simulink model "model"  (R2022a)
settings: Solver=VariableStepAuto  StartTime=0.0  StopTime=5000  RelTol=1e-3
values from neighbouring files (symbols this model uses):
  AIR_minus_delay = round(0.6/Ts)    [parameters.m]    (also in parameters.mat = 3)
  AIR_plus_delay = round(0.6/Ts)    [parameters.m]    (also in parameters.mat = 3)
  C_index = 3    [parameters.m]    (also in parameters.mat)
  C_r = 6.6    [parameters.m]    (also in parameters.mat)
  Cap_det = -1e-7    (= -1e-07)    [parameters.m]    (also in parameters.mat)
  cCap = awgn(cCap, -60)    [parameters.m]    (also in parameters.mat = [22398.4850451 24107.592632 23578.1567815 22820.4652341 2372)
  cell_count = 126    [parameters.m]    (also in parameters.mat)
  cQur = cCap / 2    [parameters.m]    (also in parameters.mat = [11880 11880 11880 11880 11880 11880 11880 11880 11880 11880)
  cTmp = 20*ones(60, 1)    [parameters.m]    (also in parameters.mat = [20 20 20 20 20 20 20 20 20 20 20 20 ... (60 elements, 60x1))
  I_CV = 1    [parameters.m]    (also in parameters.mat)
  ocv = ocv_LUT    [parameters.m]    (also in parameters.mat = [0 2.99808472822 3.29015678206 3.51449858493 3.66802196423 3)
  precharge_delay = round(0.3/Ts)    [parameters.m]    (also in parameters.mat = 1)
  Q_index = 2    [parameters.m]    (also in parameters.mat)
  R_short = 33    [parameters.m]    (also in parameters.mat)
  Rp = Rp_LUT    [parameters.m]    (also in parameters.mat = [0.0013284973182 0.00132849731829 0.00133071540687 0.0013310)
  Rs = Rs_LUT    [parameters.m]    (also in parameters.mat = [0.0044622496006 0.00446224960062 0.00395928973129 0.0036572)
  soc = soc_LUT    [parameters.m]    (also in parameters.mat = [0 0.01 0.0909090909091 0.181818181818 0.272727272727 0.3636)
  tau = tau_LUT    [parameters.m]    (also in parameters.mat = [950.87194683 950.871946837 952.459545918 952.715608142 956.)
  Ts = 0.2    [parameters.m]    (also in parameters.mat)
  U_CC = 0.06    [parameters.m]    (also in parameters.mat)
  U_sought = 4.15    [parameters.m]    (also in parameters.mat)
  U_tol = 0.0000005    (= 5e-07)    [parameters.m]    (also in parameters.mat)
undefined symbols (not defined in the file or in its folder): CC_level, CC_true, CV_level, CV_true
libraries: fl_lib x12, nesl_utility x10, simulink x3, simulink_extras x3, ee_lib x2, sharedTrackingLibrary x1
settings Model: Creator=oscar  LastModifiedBy=oscar
settings OptimizationCC: StrengthReduction=on  PassReuseOutputArgsAs=Individual arguments  ZeroExternalMemoryAtStartup=off  ZeroInternalMemoryAtStartup=off  OptimizeBlockOrder=speed  OptimizationPriority=Speed  OptimizationCustomize=off  MultiThreadedLoops=on  EfficientTunableParamExpr=on
settings DebuggingCC: ParameterTunabilityLossMsg=error  UnconnectedInputMsg=warning  UnconnectedOutputMsg=warning  UnconnectedLineMsg=warning
settings HardwareCC: ProdBitPerPointer=32  ProdBitPerSizeT=32  ProdBitPerPtrDiffT=32  ProdLargestAtomicInteger=Long  ProdLargestAtomicFloat=Double  ProdWordSize=32  ProdHWDeviceType=ARM Compatible->ARM Cortex-M
settings SFSimCC: MATLABDynamicMemAlloc=off
settings RTWCC: SystemTargetFile=ert.tlc  GenCodeOnly=on  TemplateMakefile=ert_default_tmf  GenerateReport=on  LaunchReport=on  CodeExecutionProfiling=on  DLArmComputeVersion=19.05
settings CodeAppCC: ForceParamTrailComments=on  GenerateComments=off  IgnoreCustomStorageClasses=off  OperatorAnnotations=on  SimulinkDataObjDesc=on  SFDataObjDesc=on  InsertBlockDesc=on
settings ERTTargetCC: TargetLangStandard=C99 (ISO)  CodeReplacementLibrary=ARM Cortex-M  UtilityFuncGeneration=Shared location  GenerateSampleERTMain=on  SupportComplex=off  ERTCustomFileTemplate=example_file_process.tlc

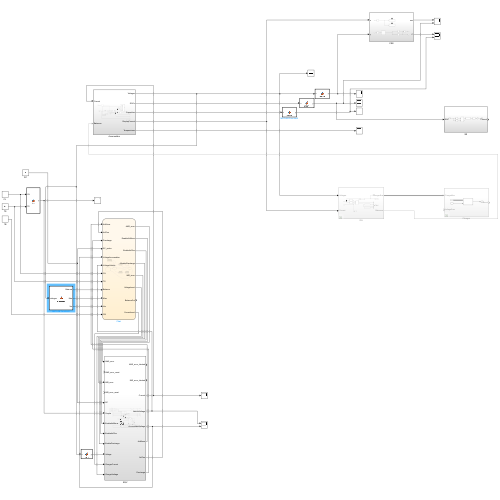
[thumbnail: Simulink's stored preview of the top-level diagram]
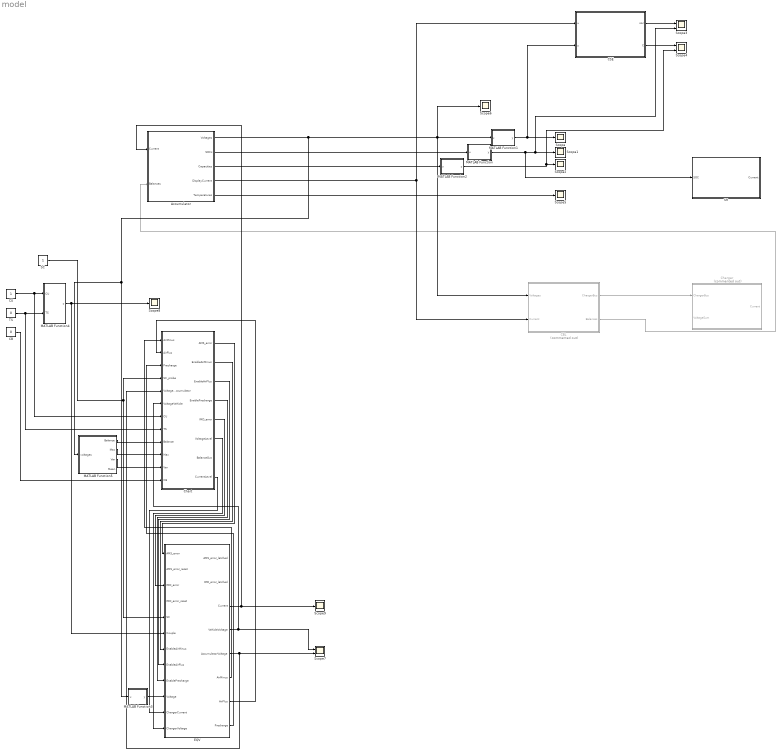
== system model ==
  Accumulator : Subsystem
  CB : Constant  Value=0
  CBL : Subsystem  Commented=on
  CSE : Subsystem
  CU : Constant
  Charger : Subsystem  Commented=on
  Chart : Stateflow chart  TreatAsAtomicUnit=on
  EQV : Subsystem
  MATLAB Function : MATLAB Function  TreatAsAtomicUnit=on
  MATLAB Function1 : MATLAB Function  TreatAsAtomicUnit=on
  MATLAB Function2 : MATLAB Function  TreatAsAtomicUnit=on
  MATLAB Function3 : MATLAB Function  TreatAsAtomicUnit=on
  MATLAB Function4 : MATLAB Function  TreatAsAtomicUnit=on
  MATLAB Function5 : MATLAB Function  TreatAsAtomicUnit=on
  SC : Constant
  SR : Subsystem
  Scope{,1..2,5..6,8..9} (7 alike) : Scope
  Scope3 : Scope  NumInputPorts=2
  Scope4 : Scope  NumInputPorts=2
  Scope7 : Scope  NumInputPorts=2
  TS : Constant  Value=0
  wires:
  Accumulator/2(SOCs) -> MATLAB Function/1(u)
  MATLAB Function/1(y) -> Scope1/1, Scope3/2, SR/1(SOC)
  MATLAB Function1/1(y) -> Scope/1, CSE/2(y)
  MATLAB Function2/1(y) -> Scope4/2, Scope2/1
  Accumulator/3(Capacities) -> MATLAB Function2/1(u)
  CBL/2(Balances) -> Accumulator/2(Balances)
  CSE/1(soc) -> Scope3/1
  CSE/2(C) -> Scope4/1
  CBL/1(ChargerBus) -> Charger/1(ChargerBus)
  Accumulator/4(DisplayCurrent) -> CSE/1(u), CBL/2(Current)
  Accumulator/5(Temperatures) -> Scope5/1
  MATLAB Function3/1(y) -> EQV/10(Voltage)
  EQV/5(AccumulatorVoltage) -> Scope7/2, Chart/5(VoltageAccumulator)
  EQV/3(Current) -> Scope9/1, Accumulator/1(Current)
  Chart/1(AMS_error) -> EQV/1(AMS_error)
  Chart/5(IMD_error) -> EQV/3(IMD_error)
  SC/1 -> EQV/5(SC), Chart/4(SC_probe)
  CU/1 -> MATLAB Function4/1(CU), Chart/7(CU)
  TS/1 -> MATLAB Function4/2(TS), Chart/8(TS)
  MATLAB Function4/1(y) -> Scope8/1, EQV/6(Couple)
  EQV/4(VehicleVoltage) -> Scope7/1, Chart/6(VoltageVehicle)
  EQV/7(AirPlus) -> Chart/2(AirPlus)
  EQV/6(AirMinus) -> Chart/1(AirMinus)
  EQV/8(Precharge) -> Chart/3(Precharge)
  Chart/4(EnablePrecharge) -> EQV/9(EnablePrecharge)
  Chart/3(EnableAirPlus) -> EQV/8(EnableAirPlus)
  Chart/2(EnableAirMinus) -> EQV/7(EnableAirMinus)
  Chart/6(VoltageLevel) -> EQV/12(ChargerVoltage)
  Accumulator/1(Voltages) -> Scope6/1, CBL/1(Voltages), MATLAB Function1/1(u), MATLAB Function5/1(voltages), MATLAB Function3/1(u)
  Chart/8(CurrentLevel) -> EQV/11(ChargerCurrent)
  MATLAB Function5/1(Balance) -> Chart/9(Balance)
  MATLAB Function5/2(Max) -> Chart/10(Max)
  MATLAB Function5/3(Var) -> Chart/11(Var)
  CB/1 -> Chart/12(CB)

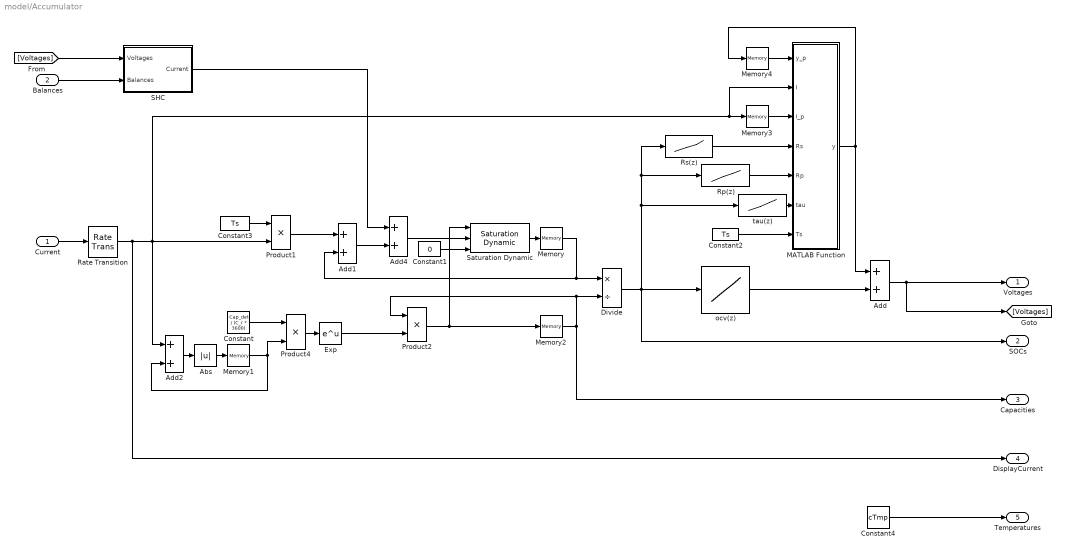
== system model/Accumulator ==
  Current : Inport
  Balances : Inport  Port=2
  Abs : Abs  SaturateOnIntegerOverflow=off
  Add{,1..2,4} (4 alike) : Sum
  Constant : Constant  Value=Cap_det / (C_r * 3600)
  Constant1 : Constant  Value=0
  Constant2 : Constant  Value=Ts
  Constant3 : Constant  Value=Ts
  Constant4 : Constant  Value=cTmp
  Divide : Product  Inputs=*/
  Exp : Math
  MATLAB Function : MATLAB Function  TreatAsAtomicUnit=on
  Memory : Memory  InitialCondition=cQur
  Memory1 : Memory
  Memory2 : Memory  InitialCondition=cCap
  Memory3 : Memory
  Memory4 : Memory  InitialCondition=zeros(cell_count, 1)
  Product1 : Product
  Product2 : Product
  Product4 : Product
  Rate Transition : RateTransition  OutPortSampleTime=Ts
  Rp(z) : Lookup_n-D  NumberOfTableDimensions=1  BreakpointsForDimension1=soc  Table=Rp  InternalRulePriority=Speed  RndMeth=Simplest
  Rs(z) : Lookup_n-D  NumberOfTableDimensions=1  BreakpointsForDimension1=soc  Table=Rs  InternalRulePriority=Speed  RndMeth=Simplest
  SHC : Subsystem
  Saturation Dynamic : simulink/Discontinuities/Saturation Dynamic  OutMin=[]  OutMax=[]  OutDataTypeStr=Inherit: Same as second input  OutDataType=fixdt(1, 16)  OutScaling=2^-10  DoSatur=off
  ocv(z) : Lookup_n-D  NumberOfTableDimensions=1  BreakpointsForDimension1=soc  Table=ocv  InternalRulePriority=Speed  RndMeth=Simplest
  tau(z) : Lookup_n-D  NumberOfTableDimensions=1  BreakpointsForDimension1=soc  Table=tau  InternalRulePriority=Speed  RndMeth=Simplest
  Voltages : Outport
  SOCs : Outport  Port=2
  Capacities : Outport  Port=3
  DisplayCurrent : Outport  Port=4
  Temperatures : Outport  Port=5
  wires:
  Constant/1 -> Product4/1
  Exp/1 -> Product2/2
  Product2/1 -> Saturation Dynamic/1, Memory2/1
  Memory1/1 -> Product4/2, Add2/2
  Abs/1 -> Memory1/1
  Memory/1 -> Divide/1, Add1/2
  Product4/1 -> Exp/1
  Add2/1 -> Abs/1
  Add/1 -> Voltages/1, [Voltages]
  Saturation Dynamic/1 -> Memory/1
  Constant1/1 -> Saturation Dynamic/3
  Memory3/1 -> MATLAB Function/3(I_p)
  tau(z)/1 -> MATLAB Function/6(tau)
  Rs(z)/1 -> MATLAB Function/4(Rs)
  Rp(z)/1 -> MATLAB Function/5(Rp)
  Memory4/1 -> MATLAB Function/1(y_p)
  MATLAB Function/1(y) -> Memory4/1, Add/1
  Constant2/1 -> MATLAB Function/7(Ts)
  Current/1 -> Rate Transition/1
  Divide/1 -> ocv(z)/1, SOCs/1, tau(z)/1, Rp(z)/1, Rs(z)/1
  Memory2/1 -> Divide/2, Product2/1, Capacities/1
  ocv(z)/1 -> Add/2
  SHC/1(Current) -> Add4/1
  Balances/1 -> SHC/2(Balances)
  Add4/1 -> Saturation Dynamic/2
  [Voltages] -> SHC/1(Voltages)
  Add1/1 -> Add4/2
  Constant4/1 -> Temperatures/1
  Constant3/1 -> Product1/1
  Rate Transition/1 -> Add2/1, Product1/2, MATLAB Function/2(I), Memory3/1, DisplayCurrent/1
  Product1/1 -> Add1/1

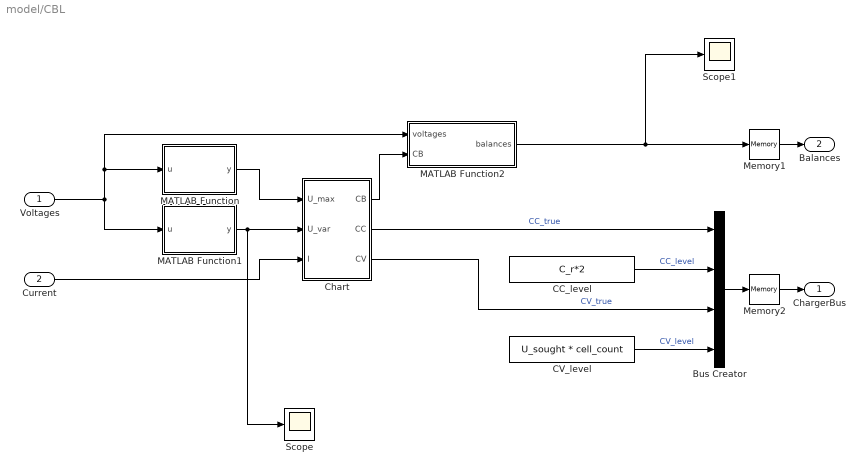
== system model/CBL ==
  Voltages : Inport
  Current : Inport  Port=2
  Bus Creator : BusCreator  Inputs=CC_true,CC_level,CV_true,CV_level
  CC_level : Constant  Value=C_r*2
  CV_level : Constant  Value=U_sought * cell_count
  Chart : Stateflow chart  TreatAsAtomicUnit=on
  MATLAB Function : MATLAB Function  TreatAsAtomicUnit=on
  MATLAB Function1 : MATLAB Function  TreatAsAtomicUnit=on
  MATLAB Function2 : MATLAB Function  TreatAsAtomicUnit=on
  Memory1 : Memory
  Memory2 : Memory
  Scope : Scope
  Scope1 : Scope
  ChargerBus : Outport
  Balances : Outport  Port=2
  wires:
  MATLAB Function/1(y) -> Chart/1(U_max)
  MATLAB Function1/1(y) -> Chart/2(U_var), Scope/1
  Voltages/1 -> MATLAB Function2/1(voltages), MATLAB Function/1(u), MATLAB Function1/1(u)
  Chart/1(CB) -> MATLAB Function2/2(CB)
  MATLAB Function2/1(balances) -> Scope1/1, Memory1/1
  Memory1/1 -> Balances/1
  Bus Creator/1 -> Memory2/1
  Current/1 -> Chart/3(I)
  CC_level/1 -> Bus Creator/2  "CC_level"
  Chart/2(CC) -> Bus Creator/1  "CC_true"
  Chart/3(CV) -> Bus Creator/3  "CV_true"
  CV_level/1 -> Bus Creator/4  "CV_level"
  Memory2/1 -> ChargerBus/1

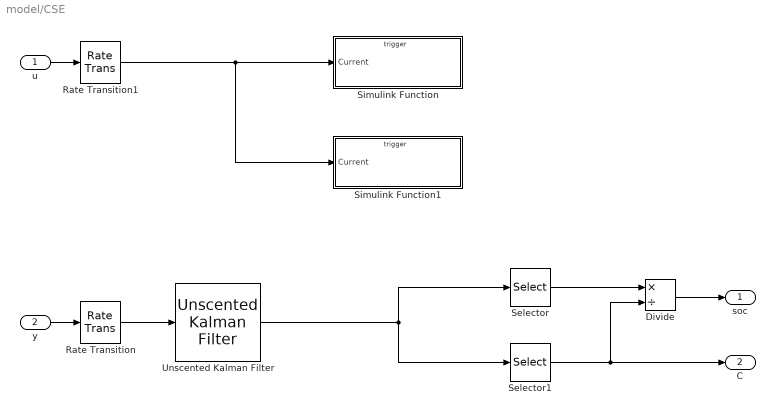
== system model/CSE ==
  u : Inport
  y : Inport  Port=2
  Divide : Product  Inputs=*/
  Rate Transition : RateTransition  OutPortSampleTime=Ts
  Rate Transition1 : RateTransition  OutPortSampleTime=Ts
  Selector : Selector  InputPortWidth=l_x  IndexOptions=Index vector (dialog)  Indices=[Q_index]  OutputSizes=1
  Selector1 : Selector  InputPortWidth=l_x  IndexOptions=Index vector (dialog)  Indices=[C_index]  OutputSizes=1
  Simulink Function : Subsystem  TreatAsAtomicUnit=on
  Simulink Function1 : Subsystem  TreatAsAtomicUnit=on
  Unscented Kalman Filter : sharedTrackingLibrary/Unscented Kalman Filter  StateTransitionFcn=S_x  HasAdditiveProcessNoise=Additive  ProcessNoise=Px0  HasTimeVaryingProcessNoise=off  HasStateTransitionFcnExtraArgument=0  InitialState=x0  InitialStateCovariance=Qx0  Alpha=1e-3  Beta=2  Kappa=0  MeasurementFcn1=M_x  HasMeasurementEnablePort1=off  HasAdditiveMeasurementNoise1=Additive  MeasurementNoise1=Rx0  HasTimeVaryingMeasurementNoise1=off  HasMeasurementFcnExtraArgument1=0  HasMeasurementWrapping1=off  MeasurementFcn2=myMeasurementFcn  HasMeasurementEnablePort2=off  HasAdditiveMeasurementNoise2=Additive  MeasurementNoise2=1  HasTimeVaryingMeasurementNoise2=off  HasMeasurementFcnExtraArgument2=0  HasMeasurementWrapping2=off  MeasurementFcn3=myMeasurementFcn  HasMeasurementEnablePort3=off  HasAdditiveMeasurementNoise3=Additive  MeasurementNoise3=1  HasTimeVaryingMeasurementNoise3=off  HasMeasurementFcnExtraArgument3=0  HasMeasurementWrapping3=off  MeasurementFcn4=myMeasurementFcn  HasMeasurementEnablePort4=off  HasAdditiveMeasurementNoise4=Additive  MeasurementNoise4=1  HasTimeVaryingMeasurementNoise4=off  HasMeasurementFcnExtraArgument4=0  HasMeasurementWrapping4=off  MeasurementFcn5=myMeasurementFcn  HasMeasurementEnablePort5=off  HasAdditiveMeasurementNoise5=Additive  MeasurementNoise5=1  HasTimeVaryingMeasurementNoise5=off  HasMeasurementFcnExtraArgument5=0  HasMeasurementWrapping5=off  EnableMultirate=off  StateTransitionFcnSampleTime=1  MeasurementFcn1SampleTime=1  MeasurementFcn2SampleTime=1  MeasurementFcn3SampleTime=1  MeasurementFcn4SampleTime=1  MeasurementFcn5SampleTime=1  UseCurrentEstimator=on  OutputStateCovariance=off  DataType=double  SampleTime=Ts  NumberOfMeasurements=1
      settings: SourceProductBaseCode=TF,AE,PW,CT,DR,ID,LP,NV,AR,RO,RR,UV,VE
  soc : Outport
  C : Outport  Port=2
  wires:
  Rate Transition/1 -> Unscented Kalman Filter/1
  Selector1/1 -> C/1, Divide/2
  Selector/1 -> Divide/1
  Divide/1 -> soc/1
  Unscented Kalman Filter/1 -> Selector1/1, Selector/1
  y/1 -> Rate Transition/1
  u/1 -> Rate Transition1/1
  Rate Transition1/1 -> Simulink Function1/1(Current), Simulink Function/1(Current)

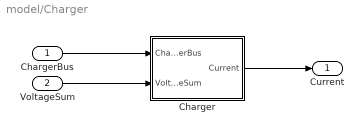
== system model/Charger ==
  ChargerBus : Inport
  VoltageSum : Inport  Port=2
  Charger : Subsystem
  Current : Outport
  wires:
  Charger/1(Current) -> Current/1
  ChargerBus/1 -> Charger/1(ChargerBus)
  VoltageSum/1 -> Charger/2(VoltageSum)

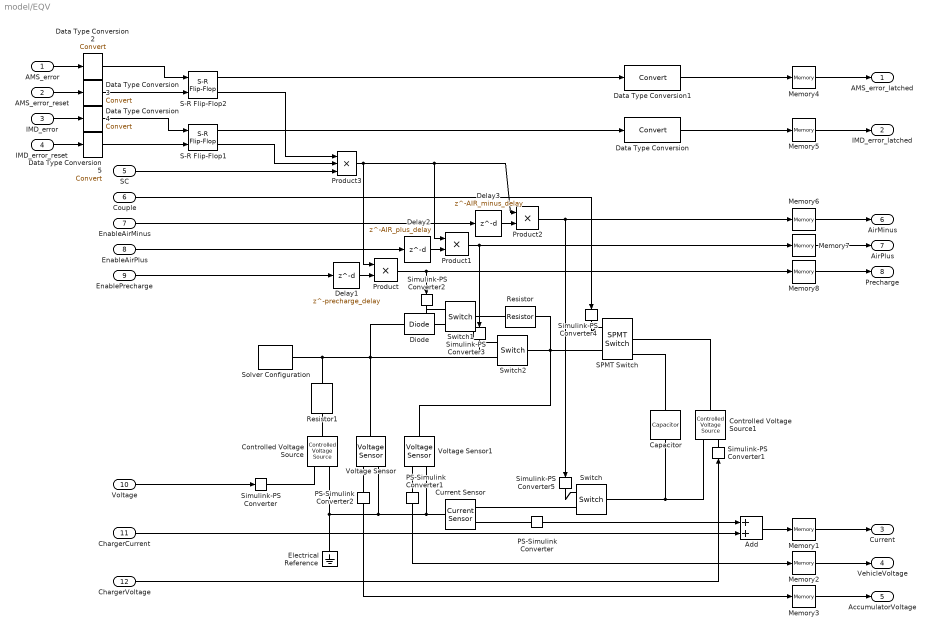
== system model/EQV ==
  AMS_error : Inport
  AMS_error_reset : Inport  Port=2
  IMD_error : Inport  Port=3
  IMD_error_reset : Inport  Port=4
  SC : Inport  Port=5
  Couple : Inport  Port=6
  EnableAirMinus : Inport  Port=7
  EnableAirPlus : Inport  Port=8
  EnablePrecharge : Inport  Port=9
  Voltage : Inport  Port=10
  ChargerCurrent : Inport  Port=11
  ChargerVoltage : Inport  Port=12
  Add : Sum
  Capacitor : fl_lib/Electrical/Electrical Elements/Capacitor  c=0.05 F  r=0 Ohm  g=1e-6 1/Ohm  i_specify=off  i_priority=None  i=0 A  i_nominal_specify=off  i_nominal_unit=A  i_nominal_value=1  v_specify=off  v_priority=None  v=0 V  v_nominal_specify=off  v_nominal_unit=V  v_nominal_value=1  vc_specify=off  vc_priority=High  vc=0 V  vc_nominal_specify=off  vc_nominal_unit=V  vc_nominal_value=1
      settings: SourceProductBaseCode=PW,SS,VE
  Controlled Voltage Source : fl_lib/Electrical/Electrical Sources/Controlled Voltage Source
      settings: SourceProductBaseCode=PW,SS,VE
  Controlled Voltage Source1 : fl_lib/Electrical/Electrical Sources/Controlled Voltage Source
      settings: SourceProductBaseCode=PW,SS,VE
  Current Sensor : fl_lib/Electrical/Electrical Sensors/Current Sensor
      settings: SourceProductBaseCode=PW,SS,VE
  Data Type Conversion{,1..5} (6 alike) : DataTypeConversion  SaturateOnIntegerOverflow=off  RndMeth=Floor
  Delay1 : Delay  DelayLength=precharge_delay  SampleTime=Ts
  Delay2 : Delay  DelayLength=AIR_plus_delay  SampleTime=Ts
  Delay3 : Delay  DelayLength=AIR_minus_delay  SampleTime=Ts
  Diode : ee_lib/Semiconductors & Converters/Diode  ModelType=ee.enum.diode.modelType.pwl  TableType=ee.enum.diode.tableType.IfMat  IfMat=[.07, .12, .19, 1.75, 4.24, 7.32, 11.2; .16, .3, .72, 2.14, 5.02, 8.35, 13.12] A  VfMat=[.9, 1.15, 1.25, 1.5, 1.75, 2.17, 2.6, 2.85; .58, .68, .75, 1.1, 1.38, 1.77, 2.27, 2.7] V  TjVec=[25, 125] degC  VfVec=[.5, .7, .9, 1.3, 1.7, 2.1, 2.5] V  IfVec=[.1, .2, .5, 1, 2, 4, 7, 10] A  Vf=0.6 V  Ron=0.3 Ohm  Goff=1e-8 S  prmExp=ee.enum.diode.expParam.useTwo  I12=[.0137, .545] A  V12=[.6, .7] V  RS=0 Ohm  Tmeas=25 degC  IS=1e-12 A  ec=1  I1=0.0137 A  V1=0.6 V  N_series=1  N_parallel=1  Rz=0.3 Ohm  BV=inf V  C_param=ee.enum.diode.capParam.fixed  CJ=5 pF  CJ0=5 pF  Vvec=[.1, 10, 100] V  Cvec=[3.5, 1, .4] pF  VJ=1 V  Mgrad=0.5  FC=0.5  Q_param=ee.enum.diode.recoveryParam.off  iRM=-7.15 A  iF=4 A  didt=-750 A/us  trr_factor=3  trr=115 ns  Qrr=150 nA*s  Vr=-600 V  Ls=150 nH  Erec=0.03 J  TT=50 ns  tau=100 ns  T_param=ee.enum.diode.temperatureParam.off  Tdevice=25 degC  I1_T2=0.245 A  V1_T2=0.5 V  IS_T2=1.25e-7 A  Tmeas2=125 degC  XTI_param=ee.enum.diode.xtiParam.pn  XTI=3  EG_param=ee.enum.diode.egapParam.material_si  EG=1.11 eV  dBVdT=0 V/K  enable_faults=simscape.enum.onoff.off  fault_action=simscape.enum.assert.action.none  fault_types=ee.enum.diode.faults.open  tau_fault=1e-3 s  IfMat_faulted=[.07, .12, .19, 1.75, 4.24, 7.32, 11.2; .16, .3, .72, 2.14, 4.02, 6.35, 9.12] A  VfMat_faulted=[.9, 1.15, 1.25, 1.5, 1.75, 2.17, 2.6, 2.85; .58, .68, .75, 1.1, 1.38, 1.77, 2.27, 2.7] V  VfVec_faulted=[.5, .7, .9, 1.3, 1.7, 2.1, 2.5] V  IfVec_faulted=[.1, .2, .5, 1, 2, 4, 7, 10] A  Ropen_faulted=1000 Ohm  Gshort_faulted=1000 1/Ohm  Vf_faulted=0.6 V  Ron_faulted=0.3 Ohm  Goff_faulted=1e-8 S  I12_faulted=[.0137, .545] A  V12_faulted=[.6, .7] V  IS_faulted=1e-12 A  ec_faulted=1  I1_faulted=0.0137 A  V1_faulted=0.6 V  RS_faulted=0 Ohm  Rz_faulted=0.3 Ohm  BV_faulted=inf V  Cscale_faulted=100  enable_temporal_fault=simscape.enum.onoff.off  t_fault=inf s  enable_behavioral_fault=simscape.enum.onoff.off  max_permissible_voltage=inf V  n_fail_on_voltage=1  max_permissible_current=inf A  t_fail_on_current=1 s  max_permissible_dVdt=inf V/s  enable_fault_input=simscape.enum.onoff.off  i_specify=off  i_priority=None  i=0 A  i_nominal_specify=off  i_nominal_unit=A  i_nominal_value=1  v_specify=off  v_priority=None  v=0 V  v_nominal_specify=off  v_nominal_unit=V  v_nominal_value=1  i_diode_specify=off  i_diode_priority=None  i_diode=0 A  i_diode_nominal_specify=off  i_diode_nominal_unit=A  i_diode_nominal_value=1  v_diode_specify=off  v_diode_priority=None  v_diode=0 V  v_diode_nominal_specify=off  v_diode_nominal_unit=V  v_diode_nominal_value=1  i_capacitor_specify=off  i_capacitor_priority=None  i_capacitor=0 A  i_capacitor_nominal_specify=off  i_capacitor_nominal_unit=A  i_capacitor_nominal_value=1  v_capacitor_specify=off  v_capacitor_priority=None  v_capacitor=0 V  v_capacitor_nominal_specify=off  v_capacitor_nominal_unit=V  v_capacitor_nominal_value=1  power_dissipated_specify=off  power_dissipated_priority=None  power_dissipated=0 W  power_dissipated_nominal_specify=off  power_dissipated_nominal_unit=W  power_dissipated_nominal_value=1  max_permissible_temperature=inf K  t_fail_on_temperature=1 s  thermal_network_parameterization=ee.enum.thermalNetworkTopology.junctionCase  Rth=[0, 10] K/W  Rth_Cauer=[1, 3, 10] K/W  Rth_Foster=[4, 6] K/W  thermal_mass_parameterization=ee.enum.thermalNetwork.timeconstant  thermal_mass=[0, 1] J/K  thermal_mass_Cauer=[.1, .3, 1] J/K  thermal_mass_Foster=[1.5, 3] J/K  thermal_time_constant=[0, 10] s  thermal_time_constant_Cauer=[1, 3, 10] s  thermal_time_constant_Foster=[6, 18] s  thermal_mass_initial_temperatures=[25, 25] degC  thermal_mass_initial_temperatures_Cauer=[25, 25, 25] degC  steadyState_Foster=simscape.enum.onoff.on  Tvec_initial_Foster=[25, 25, 25, 25] degC
  Electrical Reference : fl_lib/Electrical/Electrical Elements/Electrical Reference
      settings: SourceProductBaseCode=PW,SS,VE
  Memory{1..8} (8 alike) : Memory
  PS-Simulink Converter : nesl_utility/PS-Simulink Converter  PhysicalDomain=network_engine_domain  SubClassName=ps_output  LeftPortType=input  RightPortType=output  PseudoPeriodic=off  Frequencies=[]  VectorFormat=inherit  Unit=inherit  AffineConversion=off
      settings: SourceProductBaseCode=SS,PW,VE
  PS-Simulink Converter1 : nesl_utility/PS-Simulink Converter  PhysicalDomain=network_engine_domain  SubClassName=ps_output  LeftPortType=input  RightPortType=output  PseudoPeriodic=off  Frequencies=[]  VectorFormat=inherit  Unit=inherit  AffineConversion=off
      settings: SourceProductBaseCode=SS,PW,VE
  PS-Simulink Converter2 : nesl_utility/PS-Simulink Converter  PhysicalDomain=network_engine_domain  SubClassName=ps_output  LeftPortType=input  RightPortType=output  PseudoPeriodic=off  Frequencies=[]  VectorFormat=inherit  Unit=inherit  AffineConversion=off
      settings: SourceProductBaseCode=SS,PW,VE
  Product : Product
  Product1 : Product
  Product2 : Product
  Product3 : Product  Inputs=3
  Resistor : fl_lib/Electrical/Electrical Elements/Resistor  R=100 Ohm  i_specify=off  i_priority=None  i=0 A  i_nominal_specify=off  i_nominal_unit=A  i_nominal_value=1  v_specify=off  v_priority=None  v=0 V  v_nominal_specify=off  v_nominal_unit=V  v_nominal_value=1
      settings: SourceProductBaseCode=PW,SS,VE
  Resistor1 : fl_lib/Electrical/Electrical Elements/Resistor  R=mean(Rs)*cell_count Ohm  i_specify=off  i_priority=None  i=0 A  i_nominal_specify=off  i_nominal_unit=A  i_nominal_value=1  v_specify=off  v_priority=None  v=0 V  v_nominal_specify=off  v_nominal_unit=V  v_nominal_value=1
      settings: SourceProductBaseCode=PW,SS,VE
  S-R Flip-Flop1 : simulink_extras/Flip Flops/S-R Flip-Flop  initial_condition=0
  S-R Flip-Flop2 : simulink_extras/Flip Flops/S-R Flip-Flop  initial_condition=0
  SPMT Switch : ee_lib/Switches & Breakers/SPMT Switch  number_throws=ee.enum.switches.numberThrows.three  R_closed=0.01 Ohm  G_open=1e-6 S  enable_fault=simscape.enum.onoff.off  fault_action=simscape.enum.assert.action.none  fault_trigger=ee.enum.faults.faultTrigger.temporal  t_fault=1 s  max_permissible_current=inf A  t_fail_on_current=1 s
      settings: SourceProductBaseCode=PS  InternalSimscapePortConfiguration="{\"Bottom\":[],\"Left\":[{\"id\":\"vT\",\"label\":\"vT\",\"type\":\"input\"},{\"id\":\"p\",\"label\":\"\",\"type\":\"foundation.electrical.electrical\"}],\"Right\":[{\"id\":\"n1\",\"label\":\"\",\"type\":\"foundation.electrical.electrical\"},{\"id\":\"n2\",\"label\":\"\",\"type\":\"foundation.electrical.electrical\"},{\"id\":\"n3\",\"label\":\"\",\"type\":\"foundation.electrical.electrical\"}],\"Top\":[]}"
  Simulink-PS Converter{,1..5} (6 alike) : nesl_utility/Simulink-PS Converter  PhysicalDomain=network_engine_domain  SubClassName=ps_input  LeftPortType=input  RightPortType=output  PseudoPeriodic=off  Frequencies=[]  NoiseDistribution=none  NoiseParameters=[]  Unit=1  AffineConversion=off  FilteringAndDerivatives=provide  SimscapeFilterOrder=1  InputFilterTimeConstant=0.001  UdotUserProvided=0
      settings: SourceProductBaseCode=SS,PW,VE
  Solver Configuration : nesl_utility/Solver Configuration  PhysicalDomain=network_engine_domain  SubClassName=solver  LeftPortType=input  RightPortType=generic  Tones=[]  Harmonics=[]  SimulateNoise=off  Profile=off  UseLocalSampling=off  EnableSwitchedLinearOptims=on  FrequencyDomain=off  UseCCode=off  RelTol=0.001  AbsTol=0.001  MinStep=1e-09  ToWorkspace=off  RevertToSquareIcSolve=off  NumHomotopyIterations=100  PhasorMode=off  PhasorModeNumHarmonics=1  IndexReductionMethod=DerivativeReplacement  DoDC=off  ResidualTolerance=1e-09  UseLocalSolver=on  LocalSolverChoice=NE_BACKWARD_EULER_ADVANCER  LocalSolverSampleTime=Ts  DoFixedCost=on  MaxNonlinIter=3  MaxModeIter=2  ComputeImpulses=off  ImpulseIterations=2  LinearAlgebra=auto  LinearAlgebraNumThread=0  EquationFormulation=NE_TIME_EF  DelaysMemoryBudget=1024  AutomaticFiltering=on  FilteringTimeConstant=0.001  PartitionStorageMethod=AS_NEEDED  PartitionMemoryBudget=1024  PartitionMethod=ROBUST
      settings: SourceProductBaseCode=SS,PW,VE
  Switch : fl_lib/Electrical/Electrical Elements/Switch  R_closed=0.01 Ohm  G_open=1e-8 1/Ohm  Threshold=0.5  i_specify=off  i_priority=None  i=0 A  i_nominal_specify=off  i_nominal_unit=A  i_nominal_value=1  v_specify=off  v_priority=None  v=0 V  v_nominal_specify=off  v_nominal_unit=V  v_nominal_value=1
      settings: SourceProductBaseCode=PW,SS,VE
  Switch1 : fl_lib/Electrical/Electrical Elements/Switch  R_closed=0.01 Ohm  G_open=1e-8 1/Ohm  Threshold=0.5  i_specify=off  i_priority=None  i=0 A  i_nominal_specify=off  i_nominal_unit=A  i_nominal_value=1  v_specify=off  v_priority=None  v=0 V  v_nominal_specify=off  v_nominal_unit=V  v_nominal_value=1
      settings: SourceProductBaseCode=PW,SS,VE
  Switch2 : fl_lib/Electrical/Electrical Elements/Switch  R_closed=0.01 Ohm  G_open=1e-8 1/Ohm  Threshold=0.5  i_specify=off  i_priority=None  i=0 A  i_nominal_specify=off  i_nominal_unit=A  i_nominal_value=1  v_specify=off  v_priority=None  v=0 V  v_nominal_specify=off  v_nominal_unit=V  v_nominal_value=1
      settings: SourceProductBaseCode=PW,SS,VE
  Voltage Sensor : fl_lib/Electrical/Electrical Sensors/Voltage Sensor
      settings: SourceProductBaseCode=PW,SS,VE
  Voltage Sensor1 : fl_lib/Electrical/Electrical Sensors/Voltage Sensor
      settings: SourceProductBaseCode=PW,SS,VE
  AMS_error_latched : Outport
  IMD_error_latched : Outport  Port=2
  Current : Outport  Port=3
  VehicleVoltage : Outport  Port=4
  AccumulatorVoltage : Outport  Port=5
  AirMinus : Outport  Port=6
  AirPlus : Outport  Port=7
  Precharge : Outport  Port=8
  wires:
  EnableAirMinus/1 -> Delay3/1
  EnableAirPlus/1 -> Delay2/1
  EnablePrecharge/1 -> Delay1/1
  ChargerVoltage/1 -> Simulink-PS Converter1/1
  Memory1/1 -> Current/1
  ChargerCurrent/1 -> Add/2
  Memory3/1 -> AccumulatorVoltage/1
  PS-Simulink Converter1/1 -> Memory2/1
  Add/1 -> Memory1/1
  PS-Simulink Converter/1 -> Add/1
  PS-Simulink Converter2/1 -> Memory3/1
  Voltage/1 -> Simulink-PS Converter/1
  Memory2/1 -> VehicleVoltage/1
  Couple/1 -> Simulink-PS Converter4/1
  Product1/1 -> Memory7/1, Simulink-PS Converter3/1
  Product2/1 -> Memory6/1, Simulink-PS Converter5/1
  Product/1 -> Memory8/1, Simulink-PS Converter2/1
  Delay1/1 -> Product/2
  Delay2/1 -> Product1/2
  Delay3/1 -> Product2/2
  Product3/1 -> Product2/1, Product1/1, Product/1
  SC/1 -> Product3/3
  IMD_error_reset/1 -> Data Type Conversion5/1
  IMD_error/1 -> Data Type Conversion4/1
  AMS_error/1 -> Data Type Conversion2/1
  AMS_error_reset/1 -> Data Type Conversion3/1
  S-R Flip-Flop1/2 -> Product3/2
  S-R Flip-Flop2/2 -> Product3/1
  S-R Flip-Flop2/1 -> Data Type Conversion1/1
  S-R Flip-Flop1/1 -> Data Type Conversion/1
  Memory4/1 -> AMS_error_latched/1
  Memory5/1 -> IMD_error_latched/1
  Memory6/1 -> AirMinus/1
  Memory7/1 -> AirPlus/1
  Memory8/1 -> Precharge/1
  Data Type Conversion/1 -> Memory5/1
  Data Type Conversion1/1 -> Memory4/1
  Data Type Conversion2/1 -> S-R Flip-Flop2/1
  Data Type Conversion3/1 -> S-R Flip-Flop2/2
  Data Type Conversion4/1 -> S-R Flip-Flop1/1
  Data Type Conversion5/1 -> S-R Flip-Flop1/2
  connections:
  Controlled Voltage Source1/RConn2 -- Switch/LConn1 -- Capacitor/RConn1
  Resistor/LConn1 -- Voltage Sensor1/LConn1 -- SPMT Switch/LConn2 -- Switch2/LConn1
  Controlled Voltage Source/RConn2 -- Voltage Sensor1/RConn2 -- Current Sensor/LConn1 -- Voltage Sensor/RConn2 -- Electrical Reference/LConn1
  Resistor1/LConn1 -- Switch2/RConn2 -- Voltage Sensor/LConn1 -- Diode/LConn1 -- Solver Configuration/RConn1
  PS-Simulink Converter/LConn1 -- Current Sensor/RConn1
  Controlled Voltage Source1/LConn1 -- SPMT Switch/RConn2
  Switch1/LConn1 -- Resistor/RConn1
  Resistor1/RConn1 -- Controlled Voltage Source/LConn1
  Simulink-PS Converter1/RConn1 -- Controlled Voltage Source1/RConn1
  Switch/RConn2 -- Current Sensor/RConn2
  SPMT Switch/RConn3 -- Capacitor/LConn1
  PS-Simulink Converter1/LConn1 -- Voltage Sensor1/RConn1
  Switch1/RConn2 -- Diode/RConn1
  Simulink-PS Converter5/RConn1 -- Switch/RConn1
  Simulink-PS Converter/RConn1 -- Controlled Voltage Source/RConn1
  Simulink-PS Converter2/RConn1 -- Switch1/RConn1
  PS-Simulink Converter2/LConn1 -- Voltage Sensor/RConn1
  Simulink-PS Converter4/RConn1 -- SPMT Switch/LConn1
  Simulink-PS Converter3/RConn1 -- Switch2/RConn1

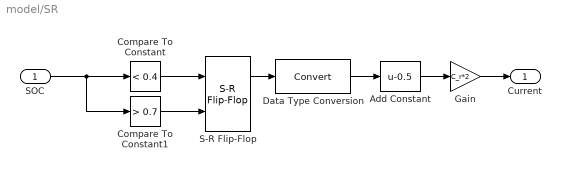
== system model/SR ==
  SOC : Inport
  Add Constant : Bias  Bias=-0.5  SaturateOnIntegerOverflow=off
  Compare To Constant : simulink/Logic and Bit Operations/Compare To Constant  relop=<  const=0.4  OutDataTypeStr=boolean
  Compare To Constant1 : simulink/Logic and Bit Operations/Compare To Constant  relop=>  const=0.7  OutDataTypeStr=boolean
  Data Type Conversion : DataTypeConversion  SaturateOnIntegerOverflow=off  RndMeth=Floor
  Gain : Gain  Gain=C_r*2
  S-R Flip-Flop : simulink_extras/Flip Flops/S-R Flip-Flop  initial_condition=0
  Current : Outport
  wires:
  Data Type Conversion/1 -> Add Constant/1
  Compare To Constant1/1 -> S-R Flip-Flop/2
  Gain/1 -> Current/1
  Add Constant/1 -> Gain/1
  S-R Flip-Flop/1 -> Data Type Conversion/1
  Compare To Constant/1 -> S-R Flip-Flop/1
  SOC/1 -> Compare To Constant1/1, Compare To Constant/1

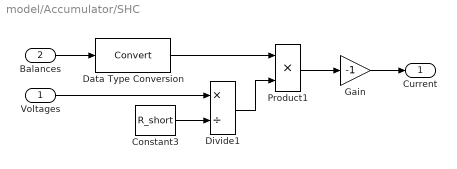
== system model/Accumulator/SHC ==
  Voltages : Inport
  Balances : Inport  Port=2
  Constant3 : Constant  Value=R_short
  Data Type Conversion : DataTypeConversion  SaturateOnIntegerOverflow=off  RndMeth=Floor
  Divide1 : Product  Inputs=*/
  Gain : Gain  Gain=-1
  Product1 : Product
  Current : Outport
  wires:
  Constant3/1 -> Divide1/2
  Data Type Conversion/1 -> Product1/1
  Divide1/1 -> Product1/2
  Balances/1 -> Data Type Conversion/1
  Product1/1 -> Gain/1
  Voltages/1 -> Divide1/1
  Gain/1 -> Current/1

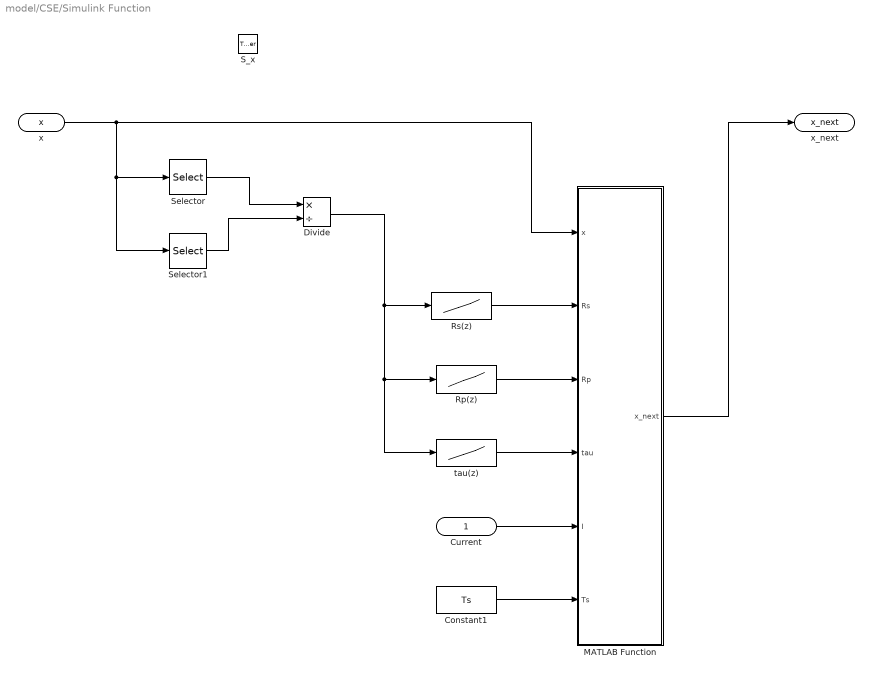
== system model/CSE/Simulink Function ==
  Current : Inport
  S_x : TriggerPort  TriggerType=function-call  IsSimulinkFunction=on  FunctionName=S_x  FunctionVisibility=scoped  VariantControl=(inherit)
  Constant1 : Constant  Value=Ts
  Divide : Product  Inputs=*/
  MATLAB Function : MATLAB Function  TreatAsAtomicUnit=on
  Rp(z) : Lookup_n-D  NumberOfTableDimensions=1  BreakpointsForDimension1=soc  Table=Rp  InternalRulePriority=Speed  RndMeth=Simplest
  Rs(z) : Lookup_n-D  NumberOfTableDimensions=1  BreakpointsForDimension1=soc  Table=Rs  InternalRulePriority=Speed  RndMeth=Simplest
  Selector : Selector  InputPortWidth=l_x  IndexOptions=Index vector (dialog)  Indices=[Q_index]  OutputSizes=1
  Selector1 : Selector  InputPortWidth=l_x  IndexOptions=Index vector (dialog)  Indices=[C_index]  OutputSizes=1
  tau(z) : Lookup_n-D  NumberOfTableDimensions=1  BreakpointsForDimension1=soc  Table=tau  InternalRulePriority=Speed  RndMeth=Simplest
  x : ArgIn  DisableCoverage=on  PortDimensions=l_x  ArgumentName=x
  x_next : ArgOut  DisableCoverage=on  PortDimensions=l_x  ArgumentName=x_next
  wires:
  Selector/1 -> Divide/1
  Rs(z)/1 -> MATLAB Function/2(Rs)
  Rp(z)/1 -> MATLAB Function/3(Rp)
  tau(z)/1 -> MATLAB Function/4(tau)
  Current/1 -> MATLAB Function/5(I)
  Constant1/1 -> MATLAB Function/6(Ts)
  MATLAB Function/1(x_next) -> x_next/1
  Selector1/1 -> Divide/2
  x/1 -> Selector1/1, Selector/1, MATLAB Function/1(x)
  Divide/1 -> Rs(z)/1, Rp(z)/1, tau(z)/1

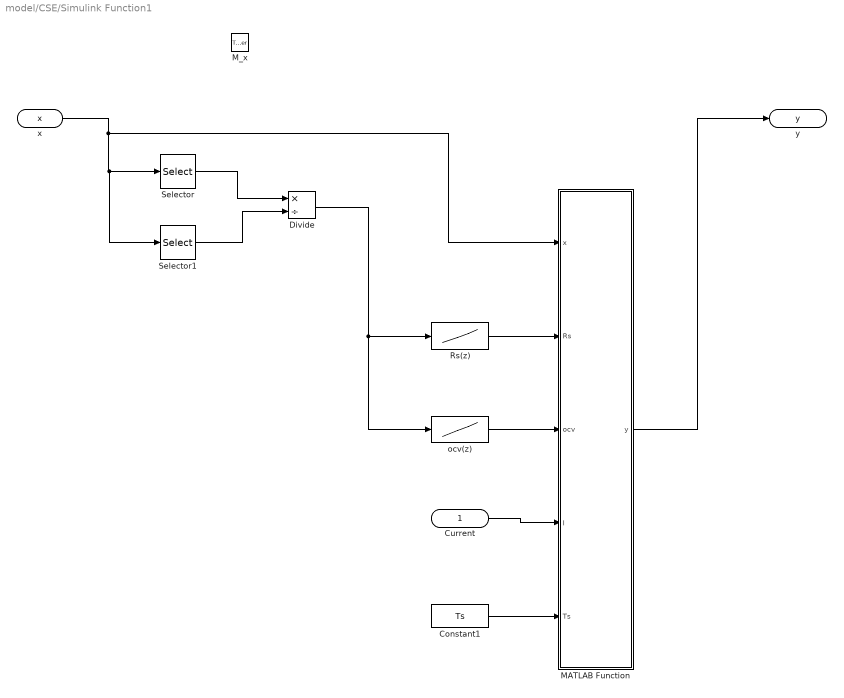
== system model/CSE/Simulink Function1 ==
  Current : Inport
  M_x : TriggerPort  TriggerType=function-call  IsSimulinkFunction=on  FunctionName=M_x  FunctionVisibility=scoped  VariantControl=(inherit)
  Constant1 : Constant  Value=Ts
  Divide : Product  Inputs=*/
  MATLAB Function : MATLAB Function  TreatAsAtomicUnit=on
  Rs(z) : Lookup_n-D  NumberOfTableDimensions=1  BreakpointsForDimension1=soc  Table=Rs  InternalRulePriority=Speed  RndMeth=Simplest
  Selector : Selector  InputPortWidth=l_x  IndexOptions=Index vector (dialog)  Indices=[Q_index]  OutputSizes=1
  Selector1 : Selector  InputPortWidth=l_x  IndexOptions=Index vector (dialog)  Indices=[C_index]  OutputSizes=1
  ocv(z) : Lookup_n-D  NumberOfTableDimensions=1  BreakpointsForDimension1=soc  Table=ocv  InternalRulePriority=Speed  RndMeth=Simplest
  x : ArgIn  DisableCoverage=on  PortDimensions=l_x  ArgumentName=x
  y : ArgOut  DisableCoverage=on  ArgumentName=y
  wires:
  Rs(z)/1 -> MATLAB Function/2(Rs)
  Current/1 -> MATLAB Function/4(I)
  MATLAB Function/1(y) -> y/1
  ocv(z)/1 -> MATLAB Function/3(ocv)
  Selector/1 -> Divide/1
  x/1 -> Selector1/1, Selector/1, MATLAB Function/1(x)
  Selector1/1 -> Divide/2
  Divide/1 -> ocv(z)/1, Rs(z)/1
  Constant1/1 -> MATLAB Function/5(Ts)

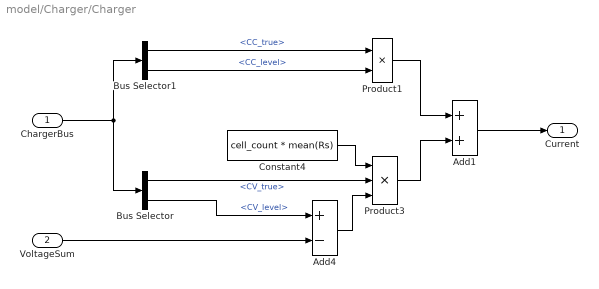
== system model/Charger/Charger ==
  ChargerBus : Inport
  VoltageSum : Inport  Port=2
  Add1 : Sum
  Add4 : Sum  Inputs=+-
  Bus Selector : BusSelector  OutputSignals=CV_true,CV_level
  Bus Selector1 : BusSelector  OutputSignals=CC_true,CC_level
  Constant4 : Constant  Value=cell_count * mean(Rs)
  Product1 : Product
  Product3 : Product  Inputs=3
  Current : Outport
  wires:
  Bus Selector/1 -> Product3/2  "<CV_true>"
  Add4/1 -> Product3/3
  VoltageSum/1 -> Add4/2
  Bus Selector/2 -> Add4/1  "<CV_level>"
  Constant4/1 -> Product3/1
  ChargerBus/1 -> Bus Selector1/1, Bus Selector/1
  Bus Selector1/1 -> Product1/1  "<CC_true>"
  Bus Selector1/2 -> Product1/2  "<CC_level>"
  Product1/1 -> Add1/1
  Product3/1 -> Add1/2
  Add1/1 -> Current/1

== matlab function model/MATLAB Function3 ==
  data: u input; y output
function y = sum(u)

y = sum(u);

== matlab function model/MATLAB Function ==
  data: u input; y output
function y = mean(u)

y = mean(u);

== matlab function model/MATLAB Function1 ==
  data: u input; y output
function y = mean(u)

y = mean(u);

== matlab function model/MATLAB Function2 ==
  data: u input; y output
function y = mean(u)

y = mean(u);

== stateflow chart model/CBL/Chart ==
  state Entry_
    CC = 0;
    CV = 0;
    CB = 0;
  state CC_state_
    CC = 1;
    CV = 0;
    CB = 0;
  state CV_state_
    CC = 0;
    CV = 1;
    CB = 0;
  state CB_state_
    CC = 0;
    CV = 0;
    CB = 1;
  (default) -> Entry_
  Entry_ -> CC_state_ [order 1] : [U_max < (U_sought - U_CC)]
  CC_state_ -> CV_state_ : [U_max > (U_sought - U_CC)]
  Entry_ -> CB_state_ [order 2] : [U_var > U_tol]
  CB_state_ -> Entry_ [order 1] : [U_var < U_tol]
  CB_state_ -> CC_state_ [order 2] : [U_max < (U_sought - U_CC)]
  CV_state_ -> CB_state_ : [I^2 < I_CV^2]
  data: U_max input; U_var input; CB output; CC output; CV output; U_CC parameter; U_tol parameter double; U_sought parameter; I_CV parameter; I input

== matlab function model/CBL/MATLAB Function ==
  data: u input; y output
function y = max(u)

y = max(u);

== matlab function model/CBL/MATLAB Function1 ==
  data: u input; y output
function y = var(u)

y = var(u);

== stateflow chart model/Chart ==
  state BalanceMode
    state Ping
      BalanceOut = Balance;
    state Pong
    (default) -> Ping
    Pong -> Ping : [after(30, sec)]
    Ping -> Pong : [after(30, sec)]
  state PrechargeDrive
    state Entry
    state CloseAirMinus
      EnableAirMinus = 1;
    state ClosePrecharge
      EnablePrecharge = 1;
    state Charge
    state CloseAirPlus
      EnableAirPlus = 1;
    state OpenPrecharge
      EnablePrecharge = 0;
    state Exit
      PrechargeDriveCplt = 1;
    state Error
      ERROR = 1
    (default) -> PrechargeDrive.Entry
    PrechargeDrive.Entry -> PrechargeDrive.CloseAirMinus
    PrechargeDrive.CloseAirMinus -> PrechargeDrive.ClosePrecharge [order 1] : [after(1, sec) && AirMinus == 1]
    PrechargeDrive.ClosePrecharge -> PrechargeDrive.Charge [order 1] : [after(1, sec) && Precharge == 1]
    PrechargeDrive.Charge -> PrechargeDrive.CloseAirPlus [order 1] : [after(1, sec) && before(45, sec) && (0.95 * VoltageAccumulator < VoltageVehicle)]
    PrechargeDrive.CloseAirPlus -> PrechargeDrive.OpenPrecharge [order 1] : [after(1, sec) && AirPlus == 1]
    PrechargeDrive.OpenPrecharge -> PrechargeDrive.Exit [order 1] : [after(1, sec) && Precharge == 0]
    PrechargeDrive.CloseAirMinus -> PrechargeDrive.Error [order 2] : [after(1.5, sec)]
    PrechargeDrive.ClosePrecharge -> PrechargeDrive.Error [order 2] : [after(1.5, sec)]
    PrechargeDrive.Charge -> PrechargeDrive.Error [order 2] : [after(45, sec)]
    PrechargeDrive.CloseAirPlus -> PrechargeDrive.Error [order 2] : [after(1.5, sec)]
    PrechargeDrive.OpenPrecharge -> PrechargeDrive.Error [order 2] : [after(1.5, sec)]
  state Drive
  state Error
    AMS_error = 1;
    IMD_error = 1;
  state Idle
  state Entry
    ERROR = 0;
    PrechargeDriveCplt = 0;
    PrechargeChargeCplt = 0;
    ChargeCplt = 0;
    EnableAirPlus = 0;
    EnableAirMinus = 0;
    BalanceOut = 0 * Balance;
  state PrechargeCharge
    state Entry
    state CloseAirMinus
      EnableAirMinus = 1;
      VoltageLevel = VoltageAccumulator;
    state ClosePrecharge
      EnablePrecharge = 1;
    state Charge
    state CloseAirPlus
      EnableAirPlus = 1;
    state OpenPrecharge
      EnablePrecharge = 0;
    state Exit
      PrechargeChargeCplt = 1;
    state Error
      ERROR = 1
    (default) -> PrechargeCharge.Entry
    PrechargeCharge.Entry -> PrechargeCharge.CloseAirMinus
    PrechargeCharge.CloseAirMinus -> PrechargeCharge.ClosePrecharge [order 1] : [after(1, sec) && AirMinus == 1]
    PrechargeCharge.ClosePrecharge -> PrechargeCharge.Charge [order 1] : [after(1, sec) && Precharge == 1]
    PrechargeCharge.Charge -> PrechargeCharge.CloseAirPlus [order 1] : [after(1, sec) && before(45, sec) && (0.95 * VoltageAccumulator < VoltageVehicle)]
    PrechargeCharge.CloseAirPlus -> PrechargeCharge.OpenPrecharge [order 1] : [after(1, sec) && AirPlus == 1]
    PrechargeCharge.OpenPrecharge -> PrechargeCharge.Exit [order 1] : [after(1, sec) && Precharge == 0]
    PrechargeCharge.CloseAirMinus -> PrechargeCharge.Error [order 2] : [after(1.5, sec)]
    PrechargeCharge.ClosePrecharge -> PrechargeCharge.Error [order 2] : [after(1.5, sec)]
    PrechargeCharge.Charge -> PrechargeCharge.Error [order 2] : [after(45, sec)]
    PrechargeCharge.CloseAirPlus -> PrechargeCharge.Error [order 2] : [after(1.5, sec)]
    PrechargeCharge.OpenPrecharge -> PrechargeCharge.Error [order 2] : [after(1.5, sec)]
  state Charge
    state Entry
    state Idle
    state CC
      CurrentLevel = 5;
      VoltageLevel = VoltageAccumulator;
      after(5, sec);
    state CV
      CurrentLevel = 0;
      VoltageLevel = 4.15 * 126;
    state Exit
      ChargeCplt = 1;
    (default) -> Charge.Entry
    Charge.Idle -> CC [order 1] : [Max < 4.14]
    Charge.Entry -> Charge.Idle
    CC -> CV : [Max > 4.14]
    CV -> Charge.Exit : [Max > 4.15]
    Charge.Idle -> Charge.Exit [order 3] : [Max > 4.15]
    Charge.Idle -> CV [order 2] : [Max > 4.0]
  BalanceMode -> Idle : [Var < 0.0001]
  Idle -> BalanceMode [order 2] : [SC_probe < 0.5 && CB > 0]
  Idle -> PrechargeDrive [order 3] : [SC_probe>0.5 && TS>0.5]
  PrechargeDrive -> Drive [order 1] : [PrechargeDriveCplt > 0.5]
  Drive -> Idle [order 2] : [TS < 0.5]
  PrechargeDrive -> Error [order 2] : [ERROR > 0.5]
  Drive -> Error [order 1] : [ERROR > 0.5]
  (default) -> Entry
  Entry -> Idle : [after(5, sec)]
  Error -> Entry
  PrechargeCharge -> Error [order 2] : [ERROR > 0.5]
  Charge -> Idle [order 1] : [CU < 0.5]
  Idle -> PrechargeCharge [order 1] : [SC_probe>0.5 && CU>0.5]
  Charge -> Error [order 2] : [ERROR > 0.5]
  PrechargeCharge -> Charge [order 1] : [PrechargeChargeCplt > 0.5]
  data: AirMinus input; AirPlus input; Precharge input; SC_probe input; VoltageAccumulator input; VoltageVehicle input; AMS_error output; EnableAirMinus output; EnableAirPlus output; EnablePrecharge output; IMD_error output; VoltageLevel output; ERROR local =0; CU input; TS input; PrechargeDriveCplt local =0; PrechargeChargeCplt local =0; Balance input; Max input; Var input; BalanceOut output; CB input; CurrentLevel output; ChargeCplt local

== matlab function model/CBL/MATLAB Function2 ==
  data: voltages input; balances output; CB input
function balances = strategy(voltages, CB)
balances = voltages*0;

if CB
    [~, I] = sort(voltages, 'descend');
    for k = 1:36
        balances(I(k)) = 1;
    end
end

== matlab function model/MATLAB Function4 ==
  data: CU input; y output; TS input
function y = fcn(CU, TS)
y = 1;
if CU
    y = 2;
elseif TS
    y = 3;
end

== matlab function model/MATLAB Function5 ==
  data: Balance output; voltages input; Max output; Var output; Mean output
function [Balance, Max, Var, Mean] = Asdasdi(voltages)

Mean = mean(voltages);
Max = max(voltages);
Var = var(voltages);
Balance = double(voltages > Mean);

== matlab function model/CSE/Simulink Function/MATLAB Function ==
  data: x input; x_next output; Rs input; Rp input; tau input; I input; Ts input
function x_next = f(x, Rs, Rp, tau, I, Ts)
x_next = zeros(3, 1);

x_next(1) = exp(-Ts / tau) * x(1) + I * (1 - exp(-Ts / tau)) * Rp;
x_next(2) = x(2) + I * Ts;
x_next(3) = x(3);
end

== matlab function model/CSE/Simulink Function1/MATLAB Function ==
  data: x input; y output; Rs input; ocv input; I input; Ts input
function y = h(x, Rs, ocv, I, Ts)

y = ocv + I * Rs + x(1);

end

== matlab function model/Accumulator/MATLAB Function ==
  data: y_p input; I input; y output; I_p input; Rs input; Rp input; tau input; Ts input
function y = mTustin(y_p, I, I_p, Rs, Rp, tau, Ts)

a = Rs.*tau;
b = Rs + Rp;
c = tau;
d = ones(length(tau), 1);

a_ = Ts*b + 2*a;
b_ = Ts*b - 2*a;
c_ = Ts*d + 2*c;
d_ = Ts*d - 2*c;

y = (a_ .*I + b_ .* I_p - d_ .* y_p) ./ c_;
